simulink model "lin_feedback2"  (R2020b)
settings: Solver=ode1  StartTime=0.0  StopTime=600  FixedStep=0.001  RelTol=1e-3  EnableMultiTasking=on
values from neighbouring files (symbols this model uses):
  cycleGain = 0.5    [advanced_model_setup.m]    (also in setup_physical.m = 1; simulate_hover.m = 0.2)
  Jp = 2*Jeq_prop    (= 0.0552224595625)    [advanced_model_setup.m]    (also in lookup_lin3d.mat; setup_lab_hover.m; setup_physical.m; simulate_hover.m)
  Jr = 2*Jeq_prop    (= 0.0552224595625)    [advanced_model_setup.m]    (also in lookup_lin3d.mat; setup_lab_hover.m; setup_physical.m; simulate_hover.m)
  K = lqi(sys, Q, R)    [gainScheduling.m]    (also in setup_lab_hover.m = K1; simulate_hover.m)
  K_AMP = 3    [advanced_model_setup.m]    (also in setup_lab_hover.m; setup_physical.m; simulate_hover.m)
  K_EC_P = 2 * pi / ( 8 * 1024 )    (= 0.000766990393943)    [advanced_model_setup.m]    (also in setup_lab_hover.m; setup_physical.m; simulate_hover.m)
  K_EC_R = 2 * pi / ( 8 * 1024 )    (= 0.000766990393943)    [advanced_model_setup.m]    (also in setup_lab_hover.m; setup_physical.m; simulate_hover.m)
  K_EC_Y = -2 * pi / ( 8 * 1024 )    (= -0.000766990393943)    [advanced_model_setup.m]    (also in setup_lab_hover.m; setup_physical.m; simulate_hover.m)
  kd = 0.5    [advanced_model_setup.m]    (also in setup_physical.m; simulate_hover.m)
  Kf = 0.1188    [advanced_model_setup.m]    (also in lookup_lin3d.mat; setup_lab_hover.m; setup_physical.m; simulate_hover.m)
  L = 7.75*0.0254    (= 0.19685)    [advanced_model_setup.m]    (also in lookup_lin3d.mat; setup_lab_hover.m; setup_physical.m; simulate_hover.m = 0.1969)
  r = 0.2    [advanced_model_setup.m]    (also in gainScheduling.m = evalin('base', 'r'); setup_physical.m = 2; simulate_hover.m = 0.5)
  skew = 1    [advanced_model_setup.m]    (also in setup_physical.m; simulate_hover.m = 2)
  V_bias = 12    [advanced_model_setup.m]    (also in setup_lab_hover.m; setup_physical.m; simulate_hover.m)
  VMAX_AMP = 24    [advanced_model_setup.m]    (also in setup_lab_hover.m; setup_physical.m; simulate_hover.m)
  wcf = 2 * pi * 20    (= 125.663706144)    [advanced_model_setup.m]    (also in setup_lab_hover.m; setup_physical.m; simulate_hover.m = 628.318530718)
  x1_traj = x1_traj*pi/180    [lookup_approxLimit.m]    (also in lookup_approxLimit3d.m)
  x1_trajectory = zeros(x1TL, x2TL)    [lookup_approxLimit.m]    (also in lookup_approxLimit3d.m = zeros(x1TL, x2TL, x3TL))
  x2_traj = x2_traj*pi/180    [lookup_approxLimit.m]    (also in lookup_approxLimit3d.m)
  x2_trajectory = zeros(x1TL, x2TL)    [lookup_approxLimit.m]    (also in lookup_approxLimit3d.m = zeros(x1TL, x2TL, x3TL))
  zetaf = 0.6    [advanced_model_setup.m]    (also in setup_lab_hover.m; setup_physical.m; simulate_hover.m)
undefined symbols (not defined in the file or in its folder): HIL, qc_get_step_size
libraries: simulink_extras x4, quarc_library x3
settings Model: SimulationMode=external  ExtModeTrigDuration=10000  Creator=hpineros  LastModifiedBy=256444
settings SolverCC: PositivePriorityOrder=on
settings DataIOCC: MaxDataPoints=5000  SaveFormat=Array  SignalLoggingSaveFormat=ModelDataLogs  InspectSignalLogs=on  ReturnWorkspaceOutputs=off
settings OptimizationCC: ExpressionDepthLimit=2147483647  InitFltsAndDblsToZero=on  LifeSpan=inf
settings DebuggingCC: SaveWithParameterizedLinksMsg=none  UnderspecifiedInitializationDetection=Classic  MergeDetectMultiDrivingBlocksExec=none  SolverPrmCheckMsg=warning  FcnCallInpInsideContextMsg=warning  StateNameClashWarn=warning  SFUnexpectedBacktrackingDiag=warning  SFNoUnconditionalDefaultTransitionDiag=warning  SFExecutionAtInitializationDiag=none  ArithmeticOperatorsInVariantConditions=warning
settings HardwareCC: ProdBitPerPointer=32  ProdBitPerSizeT=32  ProdBitPerPtrDiffT=32  ProdLargestAtomicFloat=None  ProdIntDivRoundTo=Undefined  ProdEndianess=Unspecified  ProdWordSize=32  ProdHWDeviceType=32-bit Generic
settings ModelReferenceCC: PropagateSignalLabelsOutOfModel=off
settings SFSimCC: SimUseLocalCustomCode=off  CustomCodeUndefinedFunction=UseInterfaceOnly
settings RTWCC: Description=QUARC Win64 Target  SystemTargetFile=quarc_win64.tlc  TemplateMakefile=quarc_default_tmf  RTWUseLocalCustomCode=off
settings CodeAppCC: StateflowObjectComments=on
settings STFCustomTargetCC: CombineOutputUpdateFcns=on  GRTInterface=off
settings GRTTargetCC: TargetLangStandard=C89/C90 (ANSI)  ParMdlRefBuildCompliant=off  CompOptLevelCompliant=off  MatFileLogging=off  UseToolchainInfoCompliant=off  ExtMode=on  ExtModeMexFile=quarc_comm
settings ConfigComp: CovMetricSettings=dw  CovSaveCumulativeToWorkspaceVar=on  CovSaveSingleToWorkspaceVar=on  CovExternalEMLEnable=off

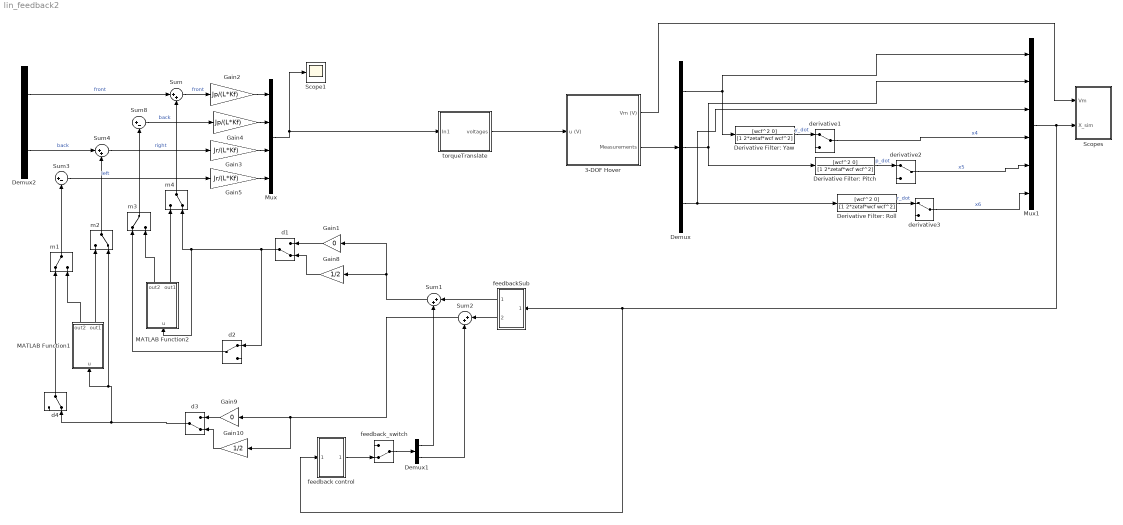
== system lin_feedback2 ==
  3-DOF Hover : Subsystem
  Demux : Demux  Outputs=3
  Demux1 : Demux  Outputs=2
  Demux2 : Demux  Outputs=2
  Derivative Filter: Pitch : TransferFcn  Numerator=[wcf^2 0]  Denominator=[1 2*zetaf*wcf wcf^2]
  Derivative Filter: Roll : TransferFcn  Numerator=[wcf^2 0]  Denominator=[1 2*zetaf*wcf wcf^2]
  Derivative Filter: Yaw : TransferFcn  Numerator=[wcf^2 0]  Denominator=[1 2*zetaf*wcf wcf^2]
  Gain1 : Gain  Gain=0
  Gain10 : Gain  Gain=1/2
  Gain2 : Gain  Gain=Jp/(L*Kf)
  Gain3 : Gain  Gain=Jr/(L*Kf)
  Gain4 : Gain  Gain=Jp/(L*Kf)
  Gain5 : Gain  Gain=Jr/(L*Kf)
  Gain8 : Gain  Gain=1/2
  Gain9 : Gain  Gain=0
  MATLAB Function1 : MATLAB Function  TreatAsAtomicUnit=on
  MATLAB Function2 : MATLAB Function  TreatAsAtomicUnit=on
  Mux : Mux
  Mux1 : Mux  Inputs=6
  Scope1 : Scope
  Scopes : Subsystem
  Sum{,1..2,4} (4 alike) : Sum  Inputs=|++
  Sum3 : Sum  Inputs=|+-
  Sum8 : Sum  Inputs=|+-
  d1 : ManualSwitch  CurrentSetting=0
  d2 : ManualSwitch
  d3 : ManualSwitch  CurrentSetting=0
  d4 : ManualSwitch  CurrentSetting=0
  derivative1 : ManualSwitch
  derivative2 : ManualSwitch
  derivative3 : ManualSwitch
  feedback control : Subsystem
  feedbackSub : Subsystem
  feedback_switch : ManualSwitch  CurrentSetting=0
  m1 : ManualSwitch
  m2 : ManualSwitch  CurrentSetting=0
  m3 : ManualSwitch
  m4 : ManualSwitch  CurrentSetting=0
  torqueTranslate : Subsystem
  wires:
  Demux/3 -> Mux1/3, Derivative Filter: Roll/1
  Demux/1 -> Mux1/1, Derivative Filter: Yaw/1
  derivative2/1 -> Mux1/5  "x5"
  derivative1/1 -> Mux1/4  "x4"
  Demux/2 -> Mux1/2, Derivative Filter: Pitch/1
  Derivative Filter: Pitch/1 -> derivative2/1  "p_dot"
  Derivative Filter: Roll/1 -> derivative3/1  "r_dot"
  Derivative Filter: Yaw/1 -> derivative1/1  "y_dot"
  3-DOF Hover/2(Measurements) -> Demux/1
  derivative3/1 -> Mux1/6  "x6"
  Mux1/1 -> feedback control/1(In1), feedbackSub/1(Input), Scopes/2(X_sim)
  3-DOF Hover/1(Vm (V)) -> Scopes/1(Vm)
  Sum/1 -> Gain2/1  "front"
  m2/1 -> Sum4/2
  Gain10/1 -> d3/2
  Sum4/1 -> Gain3/1  "right"
  d1/1 -> d2/1, m4/2, MATLAB Function2/1(u)
  MATLAB Function1/1(out2) -> m1/2
  Gain8/1 -> d1/2
  d2/1 -> m3/1
  Gain9/1 -> d3/1
  m3/1 -> Sum8/2
  m4/1 -> Sum/2
  Demux2/2 -> Sum4/1  "back"
  Gain2/1 -> Mux/1
  feedback control/1(Out1) -> feedback_switch/2
  m1/1 -> Sum3/2
  d4/1 -> m1/1
  MATLAB Function2/2(out1) -> m4/1
  Gain1/1 -> d1/1
  MATLAB Function2/1(out2) -> m3/2
  Demux2/1 -> Sum/1  "front"
  Sum3/1 -> Gain5/1  "left"
  Sum8/1 -> Gain4/1  "back"
  Gain3/1 -> Mux/3
  d3/1 -> MATLAB Function1/1(u), m2/2, d4/2
  MATLAB Function1/2(out1) -> m2/1
  Mux/1 -> Scope1/1, torqueTranslate/1(In1)
  torqueTranslate/1(voltages) -> 3-DOF Hover/1(u (V))
  feedbackSub/1(Out1) -> Sum1/1
  feedback_switch/1 -> Demux1/1
  Sum2/1 -> Gain10/1, Gain9/1
  Sum1/1 -> Gain8/1, Gain1/1
  feedbackSub/2(Out2) -> Sum2/1
  Demux1/1 -> Sum1/2
  Demux1/2 -> Sum2/2
  Gain4/1 -> Mux/2
  Gain5/1 -> Mux/4

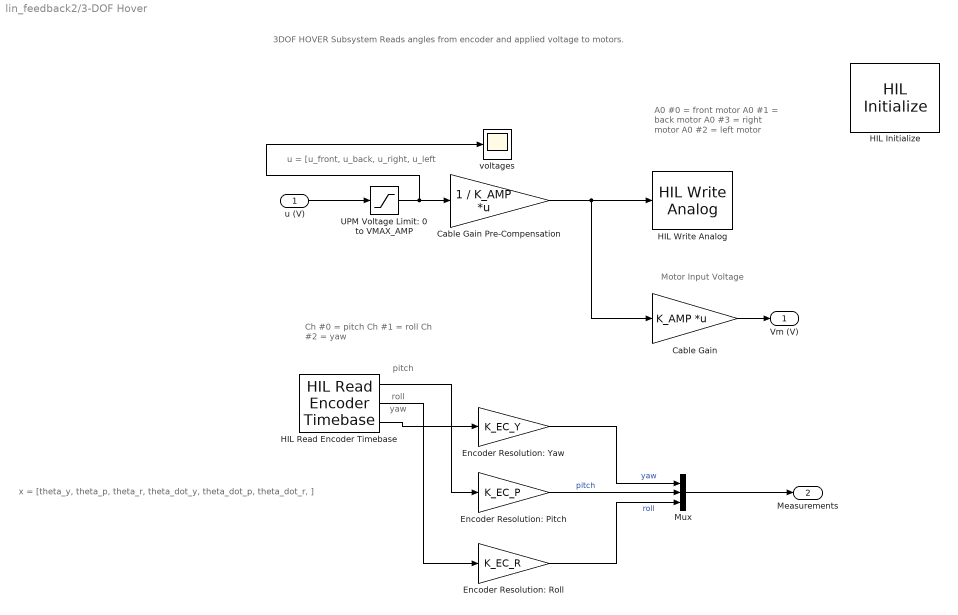
== system lin_feedback2/3-DOF Hover ==
  note: roll
  note: pitch
  note: yaw
  note: Motor Input Voltage
  note: x = [theta_y, theta_p, theta_r, theta_dot_y, theta_dot_p, theta_dot_r, ]
  note: A0 #0 = front motor
      | A0 #1 = back motor
      | A0 #3 = right motor
      | A0 #2 = left motor
  note: u = [u_front, u_back, u_right, u_left
  note: 3DOF HOVER Subsystem
      | Reads angles from encoder and applied voltage to motors.
  note: Ch #0 = pitch
      | Ch #1 = roll
      | Ch #2 = yaw
  u (V) : Inport
  Cable Gain : Gain  Gain=K_AMP  Multiplication=Matrix(K*u)  SaturateOnIntegerOverflow=on  OutDataTypeStr=Inherit: Same as input  ParamDataTypeStr=Inherit: Same as input
  Cable Gain Pre-Compensation : Gain  Gain=1 / K_AMP  Multiplication=Matrix(K*u)  SaturateOnIntegerOverflow=on  OutDataTypeStr=Inherit: Same as input  ParamDataTypeStr=Inherit: Same as input
  Encoder Resolution: Pitch : Gain  Gain=K_EC_P
  "Encoder Resolution: Roll " : Gain  Gain=K_EC_R
  Encoder Resolution: Yaw : Gain  Gain=K_EC_Y
  HIL Initialize : quarc_library/Data Acquisition/Generic/Configuration/HIL Initialize  object_name=HIL-1  board_type=q8_usb  board_number=0  board_options=update_rate=normal  exclusive=off  active=on  hardware_clocks=[0:2]  clock_modes=[]  initial_clock_frequencies=[]  set_clock_params_at_start=off  set_clock_params_at_switch_in=off  set_clock_frequencies_at_start=off  set_clock_frequencies_at_switch_in=off  analog_input_channels=[0:7]  analog_input_configurations=[]  analog_input_maximums=10  analog_input_minimums=-10  set_analog_input_params_at_start=on  set_analog_input_params_at_switch_in=off  analog_output_channels=[0:7]  analog_output_maximums=10  analog_output_minimums=-10  initial_analog_outputs=[0]  final_analog_outputs=[0]  watchdog_analog_outputs=0  set_analog_output_params_at_start=on  set_analog_output_params_at_switch_in=off  set_analog_outputs_at_start=on  set_analog_outputs_at_switch_in=off  set_analog_outputs_at_terminate=on  set_analog_outputs_at_switch_out=off  set_analog_outputs_on_watchdog=off  digital_input_channels=[]  digital_output_channels=[0:3]  digital_output_configuration=[]  initial_digital_outputs=[0]  final_digital_outputs=[0]  watchdog_digital_outputs=[0]  set_digital_output_params_at_start=off  set_digital_output_params_at_switch_in=off  set_digital_outputs_at_start=on  set_digital_outputs_at_switch_in=off  set_digital_outputs_at_terminate=on  set_digital_outputs_at_switch_out=off  set_digital_outputs_on_watchdog=off  encoder_channels=[0:7]  quadrature=[4]  encoder_filter_frequency=[]  initial_encoder_counts=[0]  set_encoder_params_at_start=on  set_encoder_params_at_switch_in=off  set_encoder_counts_at_start=on  set_encoder_counts_at_switch_in=off  pwm_channels=[0:7]  pwm_modes=0  pwm_frequency=99.532799999999995e6/4095  pwm_configuration=[0]  pwm_alignment=[0]  pwm_polarity=[1]  pwm_leading_deadband=[0]  pwm_trailing_deadband=[0]  initial_pwm_outputs=[0]  final_pwm_outputs=[0]  watchdog_pwm_outputs=[0]  set_pwm_params_at_start=on  set_pwm_params_at_switch_in=off  set_pwm_outputs_at_start=on  set_pwm_outputs_at_switch_in=off  set_pwm_outputs_at_terminate=on  set_pwm_outputs_at_switch_out=off  set_pwm_outputs_on_watchdog=off  other_output_channels=[]  initial_other_outputs=[]  final_other_outputs=[]  watchdog_other_outputs=[]  set_other_outputs_at_start=off  set_other_outputs_at_switch_in=off  set_other_outputs_at_terminate=off  set_other_outputs_at_switch_out=off  set_other_outputs_on_watchdog=off
  HIL Read Encoder Timebase : quarc_library/Data Acquisition/Generic/Timebases/HIL Read Encoder Timebase  object_name=HIL-1  clock=0  channels=[0:2]  active=on  vector_output=off  data_type_mode=Inherit via back propagation  data_type=double  overflow_mode=Error on overflow  samples_in_buffer=max(ceil(1/qc_get_step_size), 1)
  HIL Write Analog : quarc_library/Data Acquisition/Generic/Immediate I//O/HIL Write Analog  object_name=HIL-1  channels=[0,1,2,3]  sample_time=-1  active=off  vector_input=on
  Mux : Mux  Inputs=3
  UPM Voltage Limit: 0 to VMAX_AMP : Saturate  UpperLimit=VMAX_AMP  LowerLimit=0
  voltages : Scope
  Vm (V) : Outport
  Measurements : Outport  Port=2
  wires:
  Cable Gain Pre-Compensation/1 -> Cable Gain/1, HIL Write Analog/1
  HIL Read Encoder Timebase/3 -> Encoder Resolution: Yaw/1
  HIL Read Encoder Timebase/1 -> Encoder Resolution: Pitch/1
  HIL Read Encoder Timebase/2 -> "Encoder Resolution: Roll "/1
  UPM Voltage Limit: 0 to VMAX_AMP/1 -> voltages/1, Cable Gain Pre-Compensation/1
  Cable Gain/1 -> Vm (V)/1
  u (V)/1 -> UPM Voltage Limit: 0 to VMAX_AMP/1
  "Encoder Resolution: Roll "/1 -> Mux/3  "roll"
  Encoder Resolution: Yaw/1 -> Mux/1  "yaw"
  Encoder Resolution: Pitch/1 -> Mux/2  "pitch"
  Mux/1 -> Measurements/1

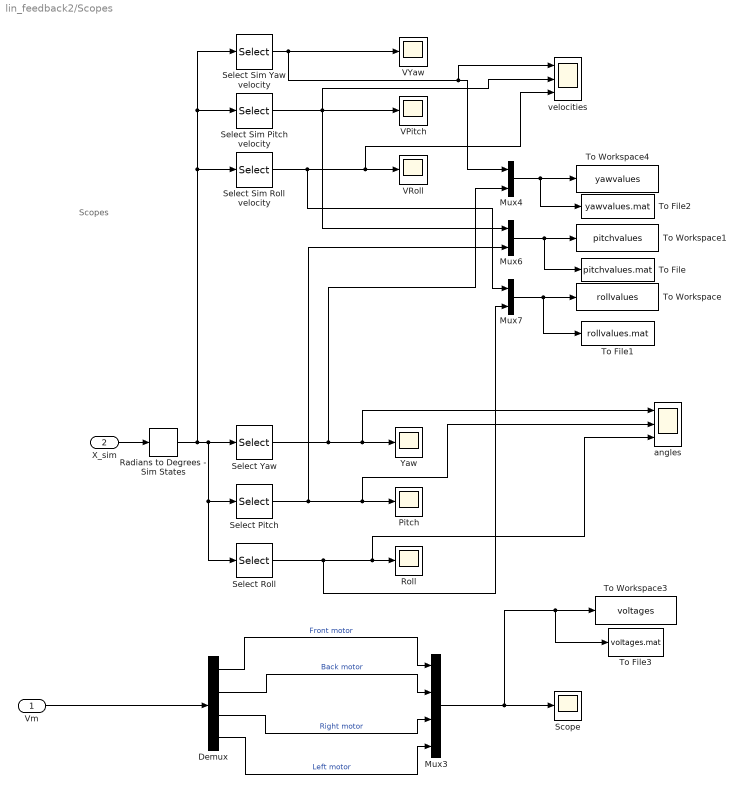
== system lin_feedback2/Scopes ==
  note: Scopes
  Vm : Inport
  X_sim : Inport  Port=2
  Demux : Demux
  Mux3 : Mux
  Mux4 : Mux  Inputs=2
  Mux6 : Mux  Inputs=2
  Mux7 : Mux  Inputs=2
  Pitch : Scope
  Radians to Degrees - Sim States : simulink_extras/Transformations/Radians to Degrees
  Roll : Scope
  Scope : Scope
  Select Pitch : Selector  InputPortWidth=6  IndexOptions=Index vector (dialog)  Indices=2  OutputSizes=1
  Select Roll : Selector  InputPortWidth=6  IndexOptions=Index vector (dialog)  Indices=3  OutputSizes=1
  Select Sim Pitch velocity : Selector  InputPortWidth=6  IndexOptions=Index vector (dialog)  Indices=5  OutputSizes=1
  Select Sim Roll velocity : Selector  InputPortWidth=6  IndexOptions=Index vector (dialog)  Indices=6  OutputSizes=1
  Select Sim Yaw velocity : Selector  InputPortWidth=6  IndexOptions=Index vector (dialog)  Indices=4  OutputSizes=1
  Select Yaw : Selector  InputPortWidth=6  IndexOptions=Index vector (dialog)  Indices=1  OutputSizes=1
  To File : ToFile  Filename=pitchvalues.mat
  To File1 : ToFile  Filename=rollvalues.mat
  To File2 : ToFile  Filename=yawvalues.mat
  To File3 : ToFile  Filename=voltages.mat
  To Workspace : ToWorkspace  VariableName=rollvalues  SampleTime=-1
  To Workspace1 : ToWorkspace  VariableName=pitchvalues  SampleTime=-1
  To Workspace3 : ToWorkspace  VariableName=voltages  SampleTime=-1
  To Workspace4 : ToWorkspace  VariableName=yawvalues  SampleTime=-1
  VPitch : Scope
  VRoll : Scope
  VYaw : Scope
  Yaw : Scope
  angles : Scope  NumInputPorts=3
  velocities : Scope  NumInputPorts=3
  wires:
  Select Roll/1 -> angles/3, Roll/1, Mux7/2
  Radians to Degrees - Sim States/1 -> Select Sim Roll velocity/1, Select Sim Pitch velocity/1, Select Sim Yaw velocity/1, Select Roll/1, Select Pitch/1, Select Yaw/1
  Select Pitch/1 -> angles/2, Pitch/1, Mux6/2
  X_sim/1 -> Radians to Degrees - Sim States/1
  Demux/1 -> Mux3/1  "Front motor"
  Demux/2 -> Mux3/2  "Back motor"
  Demux/3 -> Mux3/3  "Right motor"
  Demux/4 -> Mux3/4  "Left motor"
  Vm/1 -> Demux/1
  Select Sim Yaw velocity/1 -> VYaw/1, velocities/1, Mux4/1
  Select Sim Roll velocity/1 -> velocities/3, VRoll/1, Mux7/1
  Select Sim Pitch velocity/1 -> Mux6/1, velocities/2, VPitch/1
  Mux3/1 -> To File3/1, To Workspace3/1, Scope/1
  Select Yaw/1 -> angles/1, Yaw/1, Mux4/2
  Mux7/1 -> To File1/1, To Workspace/1
  Mux6/1 -> To File/1, To Workspace1/1
  Mux4/1 -> To File2/1, To Workspace4/1

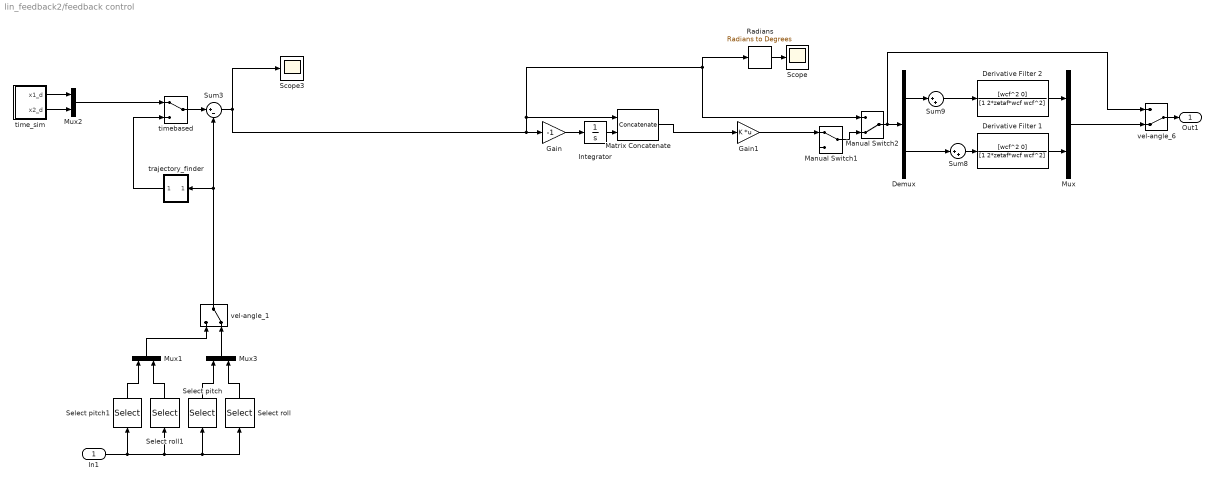
== system lin_feedback2/feedback control ==
  In1 : Inport
  Demux : Demux  Outputs=2
  Derivative Filter 1 : TransferFcn  Numerator=[wcf^2 0]  Denominator=[1 2*zetaf*wcf wcf^2]
  Derivative Filter 2 : TransferFcn  Numerator=[wcf^2 0]  Denominator=[1 2*zetaf*wcf wcf^2]
  Gain : Gain  Gain=-1
  Gain1 : Gain  Gain=K  Multiplication=Matrix(K*u)
  Integrator : Integrator
  Manual Switch1 : ManualSwitch
  Manual Switch2 : ManualSwitch  CurrentSetting=0
  Matrix Concatenate : Concatenate  Mode=Multidimensional array
  Mux{,1..3} (4 alike) : Mux  Inputs=2
  Radians : simulink_extras/Transformations/Radians to Degrees
  Scope : Scope
  Scope3 : Scope
  Select pitch : Selector  InputPortWidth=6  IndexOptions=Index vector (dialog)  Indices=2  OutputSizes=1
  Select pitch1 : Selector  InputPortWidth=6  IndexOptions=Index vector (dialog)  Indices=5  OutputSizes=1
  Select roll : Selector  InputPortWidth=6  IndexOptions=Index vector (dialog)  Indices=3  OutputSizes=1
  Select roll1 : Selector  InputPortWidth=6  IndexOptions=Index vector (dialog)  Indices=6  OutputSizes=1
  Sum3 : Sum  Inputs=|+-
  Sum8 : Sum  Inputs=|++
  Sum9 : Sum  Inputs=|++
  time_sim : Subsystem
  timebased : ManualSwitch
  trajectory_finder : Subsystem
  vel-angle_1 : ManualSwitch  CurrentSetting=0
  vel-angle_6 : ManualSwitch  CurrentSetting=0
  Out1 : Outport
  wires:
  In1/1 -> Select roll/1, Select pitch/1, Select roll1/1, Select pitch1/1
  Select pitch/1 -> Mux3/1
  time_sim/1(x1_d) -> Mux2/1
  time_sim/2(x2_d) -> Mux2/2
  Select roll/1 -> Mux3/2
  Radians/1 -> Scope/1
  Select roll1/1 -> Mux1/2
  Select pitch1/1 -> Mux1/1
  Mux1/1 -> vel-angle_1/1
  Mux3/1 -> vel-angle_1/2
  Derivative Filter 2/1 -> Mux/1
  Derivative Filter 1/1 -> Mux/2
  Manual Switch2/1 -> vel-angle_6/1, Demux/1
  vel-angle_6/1 -> Out1/1
  Demux/2 -> Sum8/1
  Mux/1 -> vel-angle_6/2
  Sum8/1 -> Derivative Filter 1/1
  Sum9/1 -> Derivative Filter 2/1
  Demux/1 -> Sum9/1
  Gain1/1 -> Manual Switch1/1
  Manual Switch1/1 -> Manual Switch2/2
  vel-angle_1/1 -> Sum3/2, trajectory_finder/1(Input)
  Sum3/1 -> Manual Switch2/1, Radians/1, Matrix Concatenate/1, Gain/1, Scope3/1
  Integrator/1 -> Matrix Concatenate/2
  Gain/1 -> Integrator/1
  timebased/1 -> Sum3/1
  Mux2/1 -> timebased/1
  trajectory_finder/1(Output) -> timebased/2
  Matrix Concatenate/1 -> Gain1/1

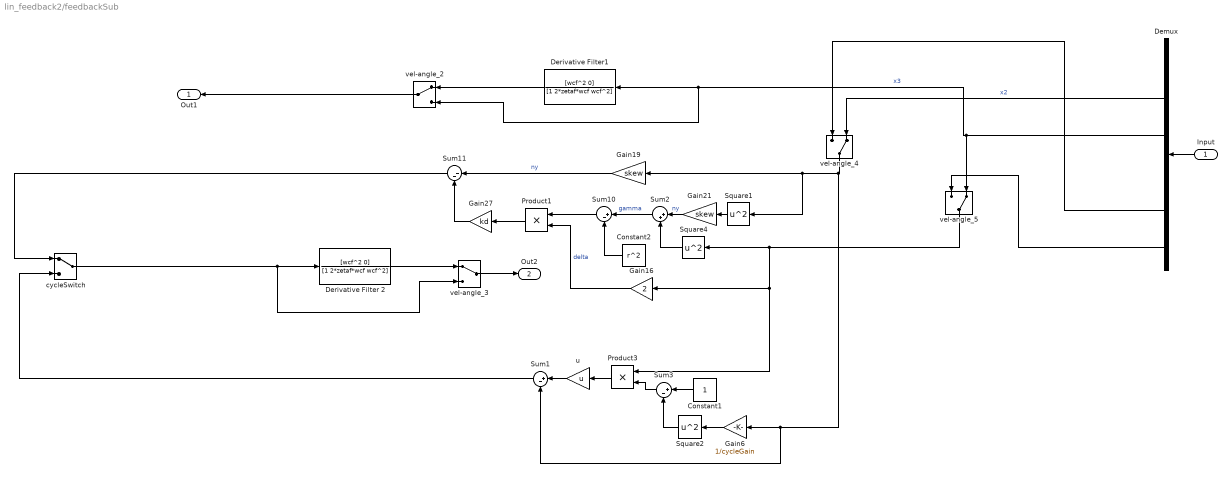
== system lin_feedback2/feedbackSub ==
  Input : Inport
  Constant1 : Constant
  Constant2 : Constant  Value=r^2
  Demux : Demux  Outputs=6
  Derivative Filter 2 : TransferFcn  Numerator=[wcf^2 0]  Denominator=[1 2*zetaf*wcf wcf^2]
  Derivative Filter1 : TransferFcn  Numerator=[wcf^2 0]  Denominator=[1 2*zetaf*wcf wcf^2]
  Gain16 : Gain  Gain=2
  Gain19 : Gain  Gain=skew
  Gain21 : Gain  Gain=skew
  Gain27 : Gain  Gain=kd
  Gain6 : Gain  Gain=1/cycleGain
  Product1 : Product
  Product3 : Product
  Square1 : Math  Operator=square  SaturateOnIntegerOverflow=on
  Square2 : Math  Operator=square  SaturateOnIntegerOverflow=on
  Square4 : Math  Operator=square  SaturateOnIntegerOverflow=on
  Sum1 : Sum  Inputs=|+-
  Sum10 : Sum  Inputs=|+-
  Sum11 : Sum  Inputs=|--
  Sum2 : Sum  Inputs=|++
  Sum3 : Sum  Inputs=|+-
  cycleSwitch : ManualSwitch
  u : Gain  Gain=u
  vel-angle_2 : ManualSwitch
  vel-angle_3 : ManualSwitch
  vel-angle_4 : ManualSwitch  CurrentSetting=0
  vel-angle_5 : ManualSwitch  CurrentSetting=0
  Out1 : Outport
  Out2 : Outport  Port=2
  wires:
  Square1/1 -> Gain21/1
  Product1/1 -> Gain27/1
  Square4/1 -> Sum2/2
  Gain19/1 -> Sum11/1  "ny"
  Sum2/1 -> Sum10/1  "gamma"
  Gain16/1 -> Product1/2  "delta"
  Sum10/1 -> Product1/1
  Gain27/1 -> Sum11/2
  Gain21/1 -> Sum2/1  "ny"
  Constant2/1 -> Sum10/2
  Sum1/1 -> cycleSwitch/2
  Demux/3 -> vel-angle_2/2, Derivative Filter1/1, vel-angle_5/2  "x3"
  u/1 -> Sum1/1
  Gain6/1 -> Square2/1
  Product3/1 -> u/1
  Constant1/1 -> Sum3/1
  Sum3/1 -> Product3/2
  Square2/1 -> Sum3/2
  Demux/2 -> vel-angle_4/2  "x2"
  Sum11/1 -> cycleSwitch/1
  Derivative Filter1/1 -> vel-angle_2/1
  vel-angle_3/1 -> Out2/1
  Derivative Filter 2/1 -> vel-angle_3/1
  Input/1 -> Demux/1
  vel-angle_4/1 -> Gain6/1, Sum1/2, Square1/1, Gain19/1
  Demux/5 -> vel-angle_4/1
  vel-angle_5/1 -> Product3/1, Gain16/1, Square4/1
  Demux/6 -> vel-angle_5/1
  cycleSwitch/1 -> vel-angle_3/2, Derivative Filter 2/1
  vel-angle_2/1 -> Out1/1

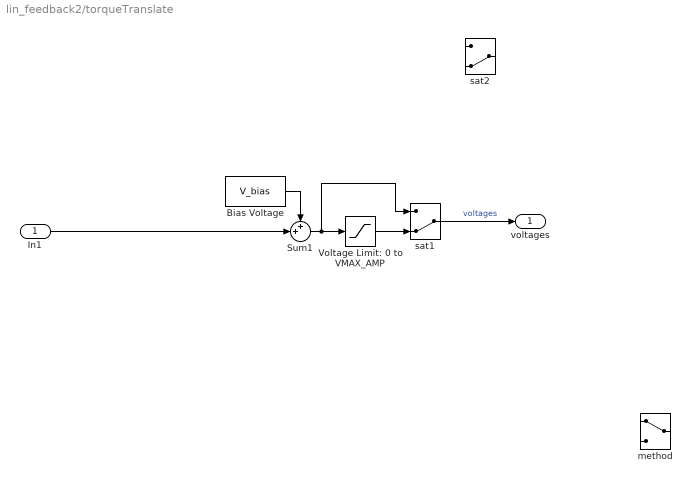
== system lin_feedback2/torqueTranslate ==
  In1 : Inport
  Bias Voltage : Constant  Value=V_bias
  Sum1 : Sum  Inputs=++|
  Voltage Limit: 0 to VMAX_AMP : Saturate  UpperLimit=VMAX_AMP  LowerLimit=0
  method : ManualSwitch
  sat1 : ManualSwitch  CurrentSetting=0
  sat2 : ManualSwitch  CurrentSetting=0
  voltages : Outport
  wires:
  Sum1/1 -> sat1/1, Voltage Limit: 0 to VMAX_AMP/1
  Voltage Limit: 0 to VMAX_AMP/1 -> sat1/2
  In1/1 -> Sum1/2
  Bias Voltage/1 -> Sum1/1
  sat1/1 -> voltages/1  "voltages"

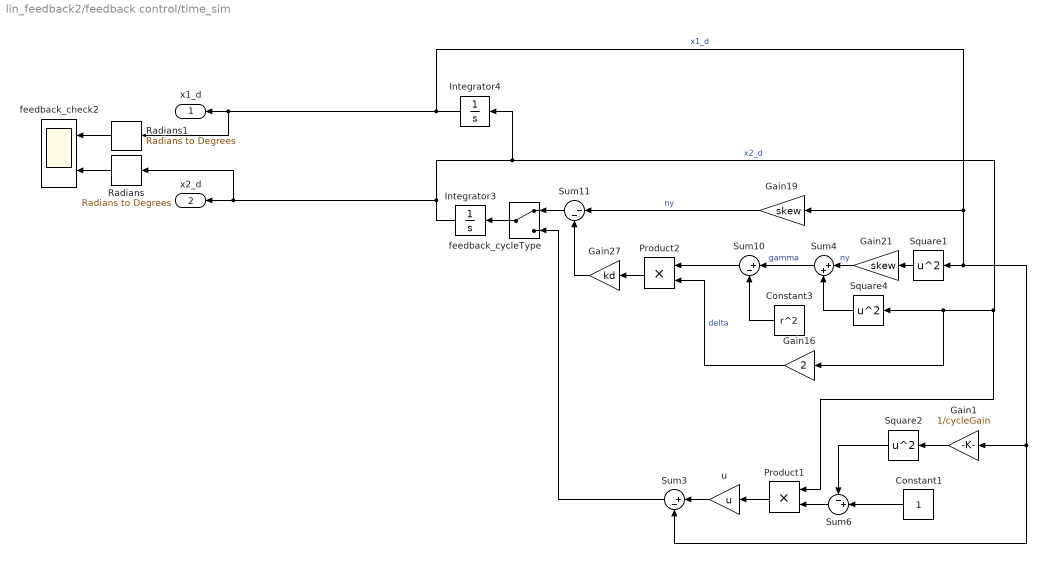
== system lin_feedback2/feedback control/time_sim ==
  Constant1 : Constant
  Constant3 : Constant  Value=r^2
  Gain1 : Gain  Gain=1/cycleGain
  Gain16 : Gain  Gain=2
  Gain19 : Gain  Gain=skew
  Gain21 : Gain  Gain=skew
  Gain27 : Gain  Gain=kd
  Integrator3 : Integrator  InitialCondition=0.00010472
  Integrator4 : Integrator  InitialCondition=0.00010472
  Product1 : Product
  Product2 : Product
  Radians : simulink_extras/Transformations/Radians to Degrees
  Radians1 : simulink_extras/Transformations/Radians to Degrees
  Square1 : Math  Operator=square  SaturateOnIntegerOverflow=on
  Square2 : Math  Operator=square  SaturateOnIntegerOverflow=on
  Square4 : Math  Operator=square  SaturateOnIntegerOverflow=on
  Sum10 : Sum  Inputs=|+-
  Sum11 : Sum  Inputs=|--
  Sum3 : Sum  Inputs=|+-
  Sum4 : Sum  Inputs=|++
  Sum6 : Sum  Inputs=-+|
  feedback_check2 : Scope  NumInputPorts=2
  feedback_cycleType : ManualSwitch
  u : Gain  Gain=u
  x1_d : Outport
  x2_d : Outport  Port=2
  wires:
  Square1/1 -> Gain21/1
  Square4/1 -> Sum4/2
  Integrator4/1 -> Sum3/2, Gain1/1, Square1/1, Gain19/1, Radians1/1, x1_d/1  "x1_d"
  Gain27/1 -> Sum11/2
  Gain16/1 -> Product2/2  "delta"
  Gain19/1 -> Sum11/1  "ny"
  Integrator3/1 -> Product1/1, Gain16/1, Square4/1, Integrator4/1, Radians/1, x2_d/1  "x2_d"
  Sum10/1 -> Product2/1
  Constant3/1 -> Sum10/2
  Gain21/1 -> Sum4/1  "ny"
  Sum4/1 -> Sum10/1  "gamma"
  Product2/1 -> Gain27/1
  Radians1/1 -> feedback_check2/1
  Radians/1 -> feedback_check2/2
  Square2/1 -> Sum6/1
  Gain1/1 -> Square2/1
  u/1 -> Sum3/1
  Product1/1 -> u/1
  Sum6/1 -> Product1/2
  Constant1/1 -> Sum6/2
  feedback_cycleType/1 -> Integrator3/1
  Sum11/1 -> feedback_cycleType/1
  Sum3/1 -> feedback_cycleType/2

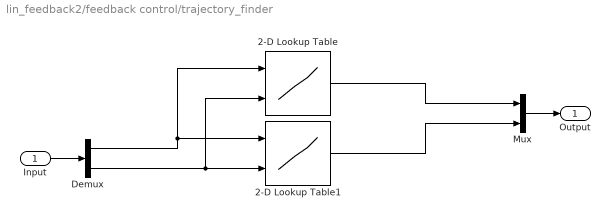
== system lin_feedback2/feedback control/trajectory_finder ==
  Input : Inport
  2-D Lookup Table : Lookup_n-D  BreakpointsForDimension1=x1_traj  BreakpointsForDimension2=x2_traj  Table=x1_trajectory  InternalRulePriority=Speed  RndMeth=Simplest  InputSameDT=on
      settings: InputPortMap=u0,u1
  2-D Lookup Table1 : Lookup_n-D  BreakpointsForDimension1=x1_traj  BreakpointsForDimension2=x2_traj  Table=x2_trajectory  InternalRulePriority=Speed  RndMeth=Simplest  InputSameDT=on
      settings: InputPortMap=u0,u1
  Demux : Demux  Outputs=2
  Mux : Mux  Inputs=2
  Output : Outport
  wires:
  2-D Lookup Table/1 -> Mux/1
  Demux/1 -> 2-D Lookup Table/1, 2-D Lookup Table1/1
  Demux/2 -> 2-D Lookup Table/2, 2-D Lookup Table1/2
  2-D Lookup Table1/1 -> Mux/2
  Mux/1 -> Output/1
  Input/1 -> Demux/1

== matlab function lin_feedback2/MATLAB Function2 ==
  data: out2 output; u input; out1 output
function [out2, out1] = fcn(u)

if u > 0
    out1 = u;
    out2 = 0;
else
    out1 = 0;
    out2 = -u;
end

== matlab function lin_feedback2/MATLAB Function1 ==
  data: out2 output; u input; out1 output
function [out2, out1] = fcn(u)

if u > 0
    out1 = u;
    out2 = 0;
else
    out1 = 0;
    out2 = -u;
end
